simulink model "NUmericalFKSimulation"  (R2021a)
settings: Solver=ode4  StartTime=0.0  StopTime=2  FixedStep=1e-3  RelTol=1e-3
values from neighbouring files (symbols this model uses):
  x_old = x(1:9)    [FKP.m]
libraries: sharedtransform x1
settings Model: Creator=Owner  LastModifiedBy=Owner

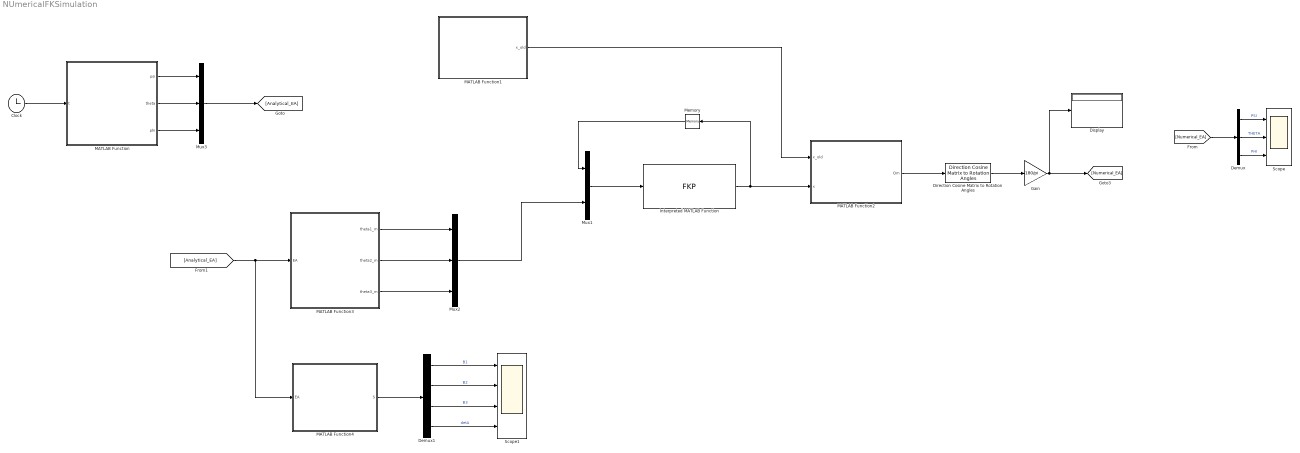
== system NUmericalFKSimulation ==
  Clock : Clock
  Demux : Demux  Outputs=3
  Demux1 : Demux
  Direction Cosine Matrix to Rotation Angles : sharedtransform/Direction Cosine Matrix to Rotation Angles  rotationOrder=ZYX  aMode=aMode  action=None  tolerance=eps(2)
      settings: SourceProductBaseCode=AE,PW,DR,MT,UV,VE
  Display : Display
  Gain : Gain  Gain=180/pi
  Interpreted MATLAB Function : MATLABFcn  MATLABFcn=FKP  OutputDimensions=9  Output1D=off
  MATLAB Function : MATLAB Function  TreatAsAtomicUnit=on
  MATLAB Function1 : MATLAB Function  TreatAsAtomicUnit=on
  MATLAB Function2 : MATLAB Function  TreatAsAtomicUnit=on
  MATLAB Function3 : MATLAB Function  TreatAsAtomicUnit=on
  MATLAB Function4 : MATLAB Function  TreatAsAtomicUnit=on
  Memory : Memory  InitialCondition=x_old
  Mux1 : Mux  Inputs=2
  Mux2 : Mux  Inputs=3
  Mux3 : Mux  Inputs=3
  Scope : Scope  NumInputPorts=3
  Scope1 : Scope  NumInputPorts=4
  wires:
  Clock/1 -> MATLAB Function/1(t)
  MATLAB Function2/1(Qm) -> Direction Cosine Matrix to Rotation Angles/1
  Direction Cosine Matrix to Rotation Angles/1 -> Gain/1
  Mux1/1 -> Interpreted MATLAB Function/1
  Interpreted MATLAB Function/1 -> Memory/1, MATLAB Function2/2(x)
  MATLAB Function3/1(theta1_m) -> Mux2/1
  MATLAB Function3/2(theta2_m) -> Mux2/2
  MATLAB Function3/3(theta3_m) -> Mux2/3
  Mux2/1 -> Mux1/2
  Memory/1 -> Mux1/1
  MATLAB Function1/1(x_old) -> MATLAB Function2/1(x_old)
  [Numerical_EA] -> Demux/1
  Gain/1 -> Display/1, [Numerical_EA]
  Demux/1 -> Scope/1  "PSI"
  Demux/2 -> Scope/2  "THETA"
  Demux/3 -> Scope/3  "PHI"
  MATLAB Function/1(psi) -> Mux3/1
  MATLAB Function/2(theta) -> Mux3/2
  MATLAB Function/3(phi) -> Mux3/3
  Mux3/1 -> [Analytical_EA]
  [Analytical_EA] -> MATLAB Function4/1(EA), MATLAB Function3/1(EA)
  MATLAB Function4/1(S) -> Demux1/1
  Demux1/2 -> Scope1/2  "B2"
  Demux1/1 -> Scope1/1  "B1"
  Demux1/3 -> Scope1/3  "B3"
  Demux1/4 -> Scope1/4  "detA"

== matlab function NUmericalFKSimulation/MATLAB Function1 ==
  data: x_old output
function x_old = InitialGuess

%% UNIT CONVERTION
dg2rd = pi/180;
rd2dg = 1/dg2rd;
mm2m = 10^(-3);
I2 = eye(2);
I3 = eye(3);
O3 = zeros(3);
I6 = eye(6);
Nm2Nmm = 1e3;

%% GEOMETRIC PARAMETERS
a1s = 65*dg2rd; sa1s = sin(a1s); ca1s = cos(a1s);
a2s = 60*dg2rd; sa2s = sin(a2s); ca2s = cos(a2s);
b1s = 0*dg2rd; sb1s = sin(b1s); cb1s = cos(b1s);
b2s = 110*dg2rd; sb2s = sin(b2s); cb2s = cos(b2s);
ETA = [0;240;120]*dg2rd;
eta1s = 0*dg2rd; se1s = sin(eta1s); ce1s = cos(eta1s);
eta2s = 240*dg2rd; se2s = sin(eta2s); ce2s = cos(eta2s);
eta3s = 120*dg2rd; se3s = sin(eta3s); ce3s = cos(eta3s);
gravity = [0;0;-9.80665];
thetaZ0 = -1.140243740887195*ones(3,1);

%% UNIT VECTORS CONSTANTS

u1v = [sb1s*se1s;sb1s*ce1s;-cb1s];
u2v = [sb1s*se2s;sb1s*ce2s;-cb1s];
u3v = [sb1s*se3s;sb1s*ce3s;-cb1s];
v1v_str = [sb2s*se1s;sb2s*ce1s;cb2s];
v2v_str = [sb2s*se2s;sb2s*ce2s;cb2s];
v3v_str = [sb2s*se3s;sb2s*ce3s;cb2s];

x_old = [v1v_str;v2v_str;v3v_str];


end

== matlab function NUmericalFKSimulation/MATLAB Function ==
  data: t input; psi output; theta output; phi output
function [psi,theta,phi] = EA_TRAJECTORY(t)



q1 = 0*(pi/180); q2 = 10*(pi/180); q3 = 10*(pi/180);

psi = q1;
theta = q2;
phi = q3;



end

== matlab function NUmericalFKSimulation/MATLAB Function2 ==
  data: x_old input; x input; Qm output
function Qm = Convert2DCM(x_old,x)


Vm_new = [x(1:3),x(4:6),x(7:9)];
Vm_OLD = [x_old(1:3),x_old(4:6),x_old(7:9)];

Qm = (Vm_new*Vm_OLD^(-1))';



end

== matlab function NUmericalFKSimulation/MATLAB Function3 ==
  data: EA input; theta1_m output; theta2_m output; theta3_m output
function [theta1_m,theta2_m,theta3_m] = INVERSE_KINEMATIC(EA)

%% UNIT CONVERTION
dg2rd = pi/180;
rd2dg = 1/dg2rd;
mm2m = 10^(-3);
I2 = eye(2);
I3 = eye(3);
O3 = zeros(3);
I6 = eye(6);
Nm2Nmm = 1e3;

%% GEOMETRIC PARAMETERS
a1s = 65*dg2rd; sa1s = sin(a1s); ca1s = cos(a1s);
a2s = 60*dg2rd; sa2s = sin(a2s); ca2s = cos(a2s);
b1s = 0*dg2rd; sb1s = sin(b1s); cb1s = cos(b1s);
b2s = 110*dg2rd; sb2s = sin(b2s); cb2s = cos(b2s);
ETA = [0;240;120]*dg2rd;
eta1s = 0*dg2rd; se1s = sin(eta1s); ce1s = cos(eta1s);
eta2s = 240*dg2rd; se2s = sin(eta2s); ce2s = cos(eta2s);
eta3s = 120*dg2rd; se3s = sin(eta3s); ce3s = cos(eta3s);
gravity = [0;0;-9.80665];
thetaZ0 = -1.140243740887195*ones(3,1);

%% UNIT VECTORS CONSTANTS

u1v = [sb1s*se1s;sb1s*ce1s;-cb1s];
u2v = [sb1s*se2s;sb1s*ce2s;-cb1s];
u3v = [sb1s*se3s;sb1s*ce3s;-cb1s];
v1v_str = [sb2s*se1s;sb2s*ce1s;cb2s];
v2v_str = [sb2s*se2s;sb2s*ce2s;cb2s];
v3v_str = [sb2s*se3s;sb2s*ce3s;cb2s];

RX= [1 0 0; 0 cos(EA(3)) -sin(EA(3)); 0 sin(EA(3)) cos(EA(3));];
RY=[cos(EA(2)) 0 sin(EA(2)); 0 1 0; -sin(EA(2)) 0 cos(EA(2));];
RZ=[cos(EA(1)) -sin(EA(1)) 0; sin(EA(1)) cos(EA(1)) 0; 0 0 1;];


Qm = RZ*RY*RX;
v1v = Qm*v1v_str;
v2v = Qm*v2v_str;
v3v = Qm*v3v_str;
%% ---LEG1----
A1_1 = sin(a1s-b1s)*(se1s*v1v(1)+ce1s*v1v(2))+cos(a1s-b1s)*v1v(3)+ca2s;
B1_1 = sa1s*(ce1s*v1v(1)-se1s*v1v(2));
C1_1 = -sin(a1s+b1s)*(se1s*v1v(1)+ce1s*v1v(2))+cos(a1s+b1s)*(v1v(3))+ca2s;
D1_1 = B1_1^2-A1_1*C1_1;
T11_1 = (-B1_1+sqrt(D1_1))/A1_1;
T12_1 = (-B1_1-sqrt(D1_1))/A1_1;
theta1_p = 2*atan(T11_1);
theta1_m = 2*atan(T12_1);
theta1 = theta1_m;

%% ---LEG2----
A2_1 = sin(a1s-b1s)*(se2s*v2v(1)+ce2s*v2v(2))+cos(a1s-b1s)*v2v(3)+ca2s;
B2_1 = sa1s*(ce2s*v2v(1)-se2s*v2v(2));
C2_1 = -sin(a1s+b1s)*(se2s*v2v(1)+ce2s*v2v(2))+cos(a1s+b1s)*(v2v(3))+ca2s;
D2_1 = B2_1^2-A2_1*C2_1;
T21_1 = (-B2_1+sqrt(D2_1))/A2_1;
T22_1 = (-B2_1-sqrt(D2_1))/A2_1;
theta2_p = 2*atan(T21_1);
theta2_m = 2*atan(T22_1);
theta2 = theta2_m;


%% ---LEG3----
A3_1 = sin(a1s-b1s)*(se3s*v3v(1)+ce3s*v3v(2))+cos(a1s-b1s)*v3v(3)+ca2s;
B3_1 = sa1s*(ce3s*v3v(1)-se3s*v3v(2));
C3_1 = -sin(a1s+b1s)*(se3s*v3v(1)+ce3s*v3v(2))+cos(a1s+b1s)*(v3v(3))+ca2s;
D3_1= B3_1^2-A3_1*C3_1;
T31_1 = (-B3_1+sqrt(D3_1))/A3_1;
T32_1 = (-B3_1-sqrt(D3_1))/A3_1;
theta3_p = 2*atan(T31_1);
theta3_m = 2*atan(T32_1);
theta3 = theta3_m;


end

== matlab function NUmericalFKSimulation/MATLAB Function4 ==
  data: EA input; S output
function S = Singulars(EA)

%% IK
%% UNIT CONVERTION
dg2rd = pi/180;
rd2dg = 1/dg2rd;
mm2m = 10^(-3);
I2 = eye(2);
I3 = eye(3);
O3 = zeros(3);
I6 = eye(6);
Nm2Nmm = 1e3;

%% GEOMETRIC PARAMETERS
a1s = 65*dg2rd; sa1s = sin(a1s); ca1s = cos(a1s);
a2s = 60*dg2rd; sa2s = sin(a2s); ca2s = cos(a2s);
b1s = 0*dg2rd; sb1s = sin(b1s); cb1s = cos(b1s);
b2s = 110*dg2rd; sb2s = sin(b2s); cb2s = cos(b2s);
ETA = [0;240;120]*dg2rd;
eta1s = 0*dg2rd; se1s = sin(eta1s); ce1s = cos(eta1s);
eta2s = 240*dg2rd; se2s = sin(eta2s); ce2s = cos(eta2s);
eta3s = 120*dg2rd; se3s = sin(eta3s); ce3s = cos(eta3s);
gravity = [0;0;-9.80665];
thetaZ0 = -1.140243740887195*ones(3,1);

%% UNIT VECTORS CONSTANTS

u1v = [sb1s*se1s;sb1s*ce1s;-cb1s];
u2v = [sb1s*se2s;sb1s*ce2s;-cb1s];
u3v = [sb1s*se3s;sb1s*ce3s;-cb1s];
v1v_str = [sb2s*se1s;sb2s*ce1s;cb2s];
v2v_str = [sb2s*se2s;sb2s*ce2s;cb2s];
v3v_str = [sb2s*se3s;sb2s*ce3s;cb2s];

RX= [1 0 0; 0 cos(EA(3)) -sin(EA(3)); 0 sin(EA(3)) cos(EA(3));];
RY=[cos(EA(2)) 0 sin(EA(2)); 0 1 0; -sin(EA(2)) 0 cos(EA(2));];
RZ=[cos(EA(1)) -sin(EA(1)) 0; sin(EA(1)) cos(EA(1)) 0; 0 0 1;];


Qm = RZ*RY*RX;
v1v = Qm*v1v_str;
v2v = Qm*v2v_str;
v3v = Qm*v3v_str;
%% ---LEG1----
A1_1 = sin(a1s-b1s)*(se1s*v1v(1)+ce1s*v1v(2))+cos(a1s-b1s)*v1v(3)+ca2s;
B1_1 = sa1s*(ce1s*v1v(1)-se1s*v1v(2));
C1_1 = -sin(a1s+b1s)*(se1s*v1v(1)+ce1s*v1v(2))+cos(a1s+b1s)*(v1v(3))+ca2s;
D1_1 = B1_1^2-A1_1*C1_1;
T11_1 = (-B1_1+sqrt(D1_1))/A1_1;
T12_1 = (-B1_1-sqrt(D1_1))/A1_1;
theta1_p = 2*atan(T11_1);
theta1_m = 2*atan(T12_1);
theta1 = theta1_m;

%% ---LEG2----
A2_1 = sin(a1s-b1s)*(se2s*v2v(1)+ce2s*v2v(2))+cos(a1s-b1s)*v2v(3)+ca2s;
B2_1 = sa1s*(ce2s*v2v(1)-se2s*v2v(2));
C2_1 = -sin(a1s+b1s)*(se2s*v2v(1)+ce2s*v2v(2))+cos(a1s+b1s)*(v2v(3))+ca2s;
D2_1 = B2_1^2-A2_1*C2_1;
T21_1 = (-B2_1+sqrt(D2_1))/A2_1;
T22_1 = (-B2_1-sqrt(D2_1))/A2_1;
theta2_p = 2*atan(T21_1);
theta2_m = 2*atan(T22_1);
theta2 = theta2_m;


%% ---LEG3----
A3_1 = sin(a1s-b1s)*(se3s*v3v(1)+ce3s*v3v(2))+cos(a1s-b1s)*v3v(3)+ca2s;
B3_1 = sa1s*(ce3s*v3v(1)-se3s*v3v(2));
C3_1 = -sin(a1s+b1s)*(se3s*v3v(1)+ce3s*v3v(2))+cos(a1s+b1s)*(v3v(3))+ca2s;
D3_1= B3_1^2-A3_1*C3_1;
T31_1 = (-B3_1+sqrt(D3_1))/A3_1;
T32_1 = (-B3_1-sqrt(D3_1))/A3_1;
theta3_p = 2*atan(T31_1);
theta3_m = 2*atan(T32_1);
theta3 = theta3_m;



%% W Vectork
THETA = [theta1_m;theta2_m;theta3_m];
theta1 = THETA(1);
theta2 = THETA(2);
theta3 = THETA(3);
w1v = [se1s*(sb1s*ca1s+cb1s*sa1s*cos(theta1))-ce1s*sa1s*sin(theta1);
       ce1s*(sb1s*ca1s+cb1s*sa1s*cos(theta1))+se1s*sa1s*sin(theta1);
       sa1s*sb1s*cos(theta1)-ca1s*cb1s
      ];
  
w2v = [se2s*(sb1s*ca1s+cb1s*sa1s*cos(theta2))-ce2s*sa1s*sin(theta2);
       ce2s*(sb1s*ca1s+cb1s*sa1s*cos(theta2))+se2s*sa1s*sin(theta2);
       sa1s*sb1s*cos(theta2)-ca1s*cb1s
      ];
  
w3v = [se3s*(sb1s*ca1s+cb1s*sa1s*cos(theta3))-ce3s*sa1s*sin(theta3);
       ce3s*(sb1s*ca1s+cb1s*sa1s*cos(theta3))+se3s*sa1s*sin(theta3);
       sa1s*sb1s*cos(theta3)-ca1s*cb1s
      ];



%% First Kind
% B1 = dot(crossVM(u1v)*w1v,v1v);
% B2 = dot(crossVM(u2v)*w2v,v2v);
% B3 = dot(crossVM(u3v)*w3v,v3v);
B1 = dot(cross(w1v,u1v),v1v);
B2 = dot(cross(w2v,u2v),v2v);
B3 = dot(cross(w3v,u3v),v3v);
FK = [B1;B2;B3];

%% Second Kind

A = [cross(w1v,v1v)';cross(w1v,v1v)';cross(w1v,v1v)'];
SK = det(A);

S = [FK;SK];

end
